simulink model "TSR_Scenario_002_cs"  (R2014b)
settings: Solver=ode5  SolverMode=SingleTasking  StartTime=0.0  StopTime=inf  FixedStep=1/100  RelTol=1e-3
PreLoadFcn:
  | mbxruntime.callbacks.PreLoadFcn(bdroot);
  | check_NUTS_defined;
  | 
  | assignin('base',['model_closed_' bdroot],false);
  | 
  | addpath('../includes_TSR/includes_TSR');
  | 
  | switch version('-release')
  | case {'2010a', '2010b', '2011a'}
  | addpath('../includes_TSR/ML2010b');
  | otherwise
  | addpath('../includes_TSR/ML2011b');
  | end
PostLoadFcn:
  | mbxruntime.callbacks.PostLoadFcn(bdroot);
InitFcn:
  | mbxruntime.callbacks.InitFcn(bdroot);;
  | 
  | addpath('..\includes_TSR');
StartFcn:
  | mbxruntime.callbacks.StartFcn(bdroot);
StopFcn:
  | mbxruntime.callbacks.StopFcn(bdroot);
model workspace: external: MAT-File .\TSR_Scenario_002_cs_hws.mat (data not in the file)
undefined symbols (not defined in the file or in its folder): InitImageOutputDir, mbxruntime, OrientationPitch, OrientationRoll, PositionX, PositionY, PositionZ, tabledata, warningInitialVelocity, x0
undefined symbols (not defined in the file): SteeringColumn, SteeringWheel, TSR_Scenario_002_cs_003e47b1b59594b6, TSR_Scenario_002_cs_023e87a31011dc74, TSR_Scenario_002_cs_048cb8409c90d9c6, TSR_Scenario_002_cs_106a0284aafa53e6, TSR_Scenario_002_cs_195b368d22a7f172, TSR_Scenario_002_cs_1e339fa5d680f213, TSR_Scenario_002_cs_26196a9fb104f950, TSR_Scenario_002_cs_261a709f6f453598, TSR_Scenario_002_cs_2ac3337370d0049d, TSR_Scenario_002_cs_2dc51e6a68b01b00, TSR_Scenario_002_cs_3460ff54d38ab2e2, TSR_Scenario_002_cs_42ea7d6e56bd6005, TSR_Scenario_002_cs_4dd419d6d2b56fc2, TSR_Scenario_002_cs_5316a21de09dff2f, TSR_Scenario_002_cs_538caacf3455966d, TSR_Scenario_002_cs_5b2cfdbcfc80811f, TSR_Scenario_002_cs_5ce0eafbb7a2dce7, TSR_Scenario_002_cs_62cdbf45c6f8824a, TSR_Scenario_002_cs_6bebc368eedff0bc, TSR_Scenario_002_cs_6d26481da4ed7e29, TSR_Scenario_002_cs_70c7e369ce6550e0, TSR_Scenario_002_cs_7a63051a1f311451, TSR_Scenario_002_cs_7d7dc8405f613c6d, TSR_Scenario_002_cs_7f65e296173485e8, TSR_Scenario_002_cs_87183cf6ff7bb4b6, TSR_Scenario_002_cs_8921b0da7ab80865, TSR_Scenario_002_cs_9495ce3a76763d1f, TSR_Scenario_002_cs_a679806a2fdc8099, TSR_Scenario_002_cs_Actros_1860_1_Path_pathUniqueID, TSR_Scenario_002_cs_Actros_2541_1_Path_pathUniqueID, TSR_Scenario_002_cs_Actros_2541_3_Path_pathUniqueID, TSR_Scenario_002_cs_Actros_2541_4_Path_pathUniqueID, TSR_Scenario_002_cs_adf24c93a9de8a4e, TSR_Scenario_002_cs_Audi_A8_1_Dynamics_Simple_initialPitch, TSR_Scenario_002_cs_Audi_A8_1_Dynamics_Simple_initialRoll, TSR_Scenario_002_cs_Audi_A8_1_Dynamics_Simple_initialX, TSR_Scenario_002_cs_Audi_A8_1_Dynamics_Simple_initialY, TSR_Scenario_002_cs_Audi_A8_1_Dynamics_Simple_initialYaw, TSR_Scenario_002_cs_Audi_A8_1_Dynamics_Simple_initialZ, TSR_Scenario_002_cs_b136c6ccb55f77db, TSR_Scenario_002_cs_ba4f809714c282b7, TSR_Scenario_002_cs_BMW_X5_1_Path_pathUniqueID, TSR_Scenario_002_cs_BMW_X5_1_SpeedProfile_speedProfileUniqueID, TSR_Scenario_002_cs_BMW_X5_2_Path_pathUniqueID, TSR_Scenario_002_cs_BMW_X5_2_SpeedProfile_speedProfileUniqueID, TSR_Scenario_002_cs_Citroen_C3_1_Path_pathUniqueID, TSR_Scenario_002_cs_Citroen_C3_2_Path_pathUniqueID, TSR_Scenario_002_cs_d8f275339b7082cf, TSR_Scenario_002_cs_Daf_95_1_Path_pathUniqueID, TSR_Scenario_002_cs_Daf_95_1_SpeedProfile_speedProfileUniqueID, TSR_Scenario_002_cs_dc019741510ce2f2, TSR_Scenario_002_cs_fdbc8aabe460b27c, TSR_Scenario_002_cs_Fiat_Bravo_1_Path_pathUniqueID, TSR_Scenario_002_cs_Ford_Fiesta_1_Path_pathUniqueID, TSR_Scenario_002_cs_Honda_Pan_European_1_Path_pathUniqueID, TSR_Scenario_002_cs_Mazda_RX8_1_Path_pathUniqueID, TSR_Scenario_002_cs_Nissan_Cabstar_1_Path_pathUniqueID, TSR_Scenario_002_cs_Nissan_Cabstar_2_Path_pathUniqueID ... (+9)
libraries: simulink_extras x82, simulink x23, PreScanSimulinkLibrary x11
(part 10 of 39)

== system TSR_Scenario_002_cs/HighwayOverhang_11 ==
  note: Resources
      |
      | 1: InformationSign\MatrixSign_GreenArrow.png: MatrixSign GreenArrow
      | 2: InformationSign\Empty.jpeg: Empty
      | 3: InformationSign\SEARCH_Logo.png: SEARCH Logo
      | 4: InformationSign\z274-50_black_full.png: z274-50 black full
      | 5: InformationSign\z274-51_black_full.png: z274-51 black full
      | 6: InformationSign\z274-52_black_full.png: z274-52 black full
      | 7: InformationSign\z274-53_black_full.png: z274-53 black full
      | 8: InformationSign\z274-54_black_full.png: z274-54 black full
      | 9: InformationSign\z274-55_black_full.png: z274-55 black full
      | 10: InformationSign\z274-56_black_full.png: z274-56 black full
      | 11: InformationSign\z274-57_black_full.png: z274-57 black full
      | 12: InformationSign\z274-58_black_full.png: z274-58 black full
      | 13: InformationSign\z274-59_black_full.png: z274-59 black full
      | 14: InformationSign\z274-60_black_full.png: z274-60 black full
      | 15: InformationSign\z274-61_black_full.png: z274-61 black full
      | 16: InformationSign\z274-62_black_full.png: z274-62 black full
      | 17: InformationSign\z274-63_black_full.png: z274-63 black full
  Ground_{1..4} (4 alike) : Ground
  VISUMatrixSignLights_Mux : Subsystem  Tag=mux/VisuMatrixSignLights  mask(PreScan User Interface: VisuMatrixSignLights){}
      mask help:
      | The VisuMatrixSignLights block provides a way to switch the lights on the matrix sign board on or off
      |
      | For more information, please click Help.
      mask Help: eval('openHelp(732)')
  VISUMatrixSign_Mux : Subsystem  Tag=mux/MatrixSign_v2  mask(PreScan User Interface: VisuMatrixSign){}
      mask help:
      | The VisuMatrixSign block provides a way to adapt the texture of the plates connected to an overhang, based on Resource IDs of the texture files.
      |
      | For more information, please click Help.
      settings: DeleteFcn=PreScanBlockDeleteFcn;
      mask Help: eval('openHelp(733)')
  VISUMatrixSign_HighwayOverhang_11 : Outport  Tag=outport/VisuMatrixSign  SampleTime=1/100
  VISUMatrixSignLights_HighwayOverhang_11 : Outport  Tag=outport/VisuMatrixSignLights  Port=2  SampleTime=1/100
  wires:
  VISUMatrixSign_Mux/1(MatrixSigns) -> VISUMatrixSign_HighwayOverhang_11/1
  VISUMatrixSignLights_Mux/1(VISUMatrixSignLights_HighwayOverhang_11) -> VISUMatrixSignLights_HighwayOverhang_11/1
  Ground_1/1 -> VISUMatrixSignLights_Mux/1(MatrixSign_10)
  Ground_2/1 -> VISUMatrixSignLights_Mux/2(MatrixSign_49)
  Ground_3/1 -> VISUMatrixSign_Mux/1(MatrixSign_10)
  Ground_4/1 -> VISUMatrixSign_Mux/2(MatrixSign_49)

== system TSR_Scenario_002_cs/HighwayOverhang_12 ==
  note: Resources
      |
      | 1: InformationSign\MatrixSign_GreenArrow.png: MatrixSign GreenArrow
      | 2: InformationSign\Empty.jpeg: Empty
      | 3: InformationSign\SEARCH_Logo.png: SEARCH Logo
      | 4: InformationSign\z274-50_black_full.png: z274-50 black full
      | 5: InformationSign\z274-51_black_full.png: z274-51 black full
      | 6: InformationSign\z274-52_black_full.png: z274-52 black full
      | 7: InformationSign\z274-53_black_full.png: z274-53 black full
      | 8: InformationSign\z274-54_black_full.png: z274-54 black full
      | 9: InformationSign\z274-55_black_full.png: z274-55 black full
      | 10: InformationSign\z274-56_black_full.png: z274-56 black full
      | 11: InformationSign\z274-57_black_full.png: z274-57 black full
      | 12: InformationSign\z274-58_black_full.png: z274-58 black full
      | 13: InformationSign\z274-59_black_full.png: z274-59 black full
      | 14: InformationSign\z274-60_black_full.png: z274-60 black full
      | 15: InformationSign\z274-61_black_full.png: z274-61 black full
      | 16: InformationSign\z274-62_black_full.png: z274-62 black full
      | 17: InformationSign\z274-63_black_full.png: z274-63 black full
  Ground_{1..4} (4 alike) : Ground
  VISUMatrixSignLights_Mux : Subsystem  Tag=mux/VisuMatrixSignLights  mask(PreScan User Interface: VisuMatrixSignLights){}
      mask help:
      | The VisuMatrixSignLights block provides a way to switch the lights on the matrix sign board on or off
      |
      | For more information, please click Help.
      mask Help: eval('openHelp(732)')
  VISUMatrixSign_Mux : Subsystem  Tag=mux/MatrixSign_v2  mask(PreScan User Interface: VisuMatrixSign){}
      mask help:
      | The VisuMatrixSign block provides a way to adapt the texture of the plates connected to an overhang, based on Resource IDs of the texture files.
      |
      | For more information, please click Help.
      settings: DeleteFcn=PreScanBlockDeleteFcn;
      mask Help: eval('openHelp(733)')
  VISUMatrixSign_HighwayOverhang_12 : Outport  Tag=outport/VisuMatrixSign  SampleTime=1/100
  VISUMatrixSignLights_HighwayOverhang_12 : Outport  Tag=outport/VisuMatrixSignLights  Port=2  SampleTime=1/100
  wires:
  VISUMatrixSign_Mux/1(MatrixSigns) -> VISUMatrixSign_HighwayOverhang_12/1
  VISUMatrixSignLights_Mux/1(VISUMatrixSignLights_HighwayOverhang_12) -> VISUMatrixSignLights_HighwayOverhang_12/1
  Ground_1/1 -> VISUMatrixSignLights_Mux/1(MatrixSign_21)
  Ground_2/1 -> VISUMatrixSignLights_Mux/2(MatrixSign_22)
  Ground_3/1 -> VISUMatrixSign_Mux/1(MatrixSign_21)
  Ground_4/1 -> VISUMatrixSign_Mux/2(MatrixSign_22)

== system TSR_Scenario_002_cs/HighwayOverhang_13 ==
  note: Resources
      |
      | 1: InformationSign\MatrixSign_GreenArrow.png: MatrixSign GreenArrow
      | 2: InformationSign\Empty.jpeg: Empty
      | 3: InformationSign\SEARCH_Logo.png: SEARCH Logo
      | 4: InformationSign\z274-50_black_full.png: z274-50 black full
      | 5: InformationSign\z274-51_black_full.png: z274-51 black full
      | 6: InformationSign\z274-52_black_full.png: z274-52 black full
      | 7: InformationSign\z274-53_black_full.png: z274-53 black full
      | 8: InformationSign\z274-54_black_full.png: z274-54 black full
      | 9: InformationSign\z274-55_black_full.png: z274-55 black full
      | 10: InformationSign\z274-56_black_full.png: z274-56 black full
      | 11: InformationSign\z274-57_black_full.png: z274-57 black full
      | 12: InformationSign\z274-58_black_full.png: z274-58 black full
      | 13: InformationSign\z274-59_black_full.png: z274-59 black full
      | 14: InformationSign\z274-60_black_full.png: z274-60 black full
      | 15: InformationSign\z274-61_black_full.png: z274-61 black full
      | 16: InformationSign\z274-62_black_full.png: z274-62 black full
      | 17: InformationSign\z274-63_black_full.png: z274-63 black full
  Ground_{1..4} (4 alike) : Ground
  VISUMatrixSignLights_Mux : Subsystem  Tag=mux/VisuMatrixSignLights  mask(PreScan User Interface: VisuMatrixSignLights){}
      mask help:
      | The VisuMatrixSignLights block provides a way to switch the lights on the matrix sign board on or off
      |
      | For more information, please click Help.
      mask Help: eval('openHelp(732)')
  VISUMatrixSign_Mux : Subsystem  Tag=mux/MatrixSign_v2  mask(PreScan User Interface: VisuMatrixSign){}
      mask help:
      | The VisuMatrixSign block provides a way to adapt the texture of the plates connected to an overhang, based on Resource IDs of the texture files.
      |
      | For more information, please click Help.
      settings: DeleteFcn=PreScanBlockDeleteFcn;
      mask Help: eval('openHelp(733)')
  VISUMatrixSign_HighwayOverhang_13 : Outport  Tag=outport/VisuMatrixSign  SampleTime=1/100
  VISUMatrixSignLights_HighwayOverhang_13 : Outport  Tag=outport/VisuMatrixSignLights  Port=2  SampleTime=1/100
  wires:
  VISUMatrixSign_Mux/1(MatrixSigns) -> VISUMatrixSign_HighwayOverhang_13/1
  VISUMatrixSignLights_Mux/1(VISUMatrixSignLights_HighwayOverhang_13) -> VISUMatrixSignLights_HighwayOverhang_13/1
  Ground_1/1 -> VISUMatrixSignLights_Mux/1(MatrixSign_3)
  Ground_2/1 -> VISUMatrixSignLights_Mux/2(MatrixSign_44)
  Ground_3/1 -> VISUMatrixSign_Mux/1(MatrixSign_3)
  Ground_4/1 -> VISUMatrixSign_Mux/2(MatrixSign_44)

== system TSR_Scenario_002_cs/HighwayOverhang_14 ==
  note: Resources
      |
      | 1: InformationSign\MatrixSign_GreenArrow.png: MatrixSign GreenArrow
      | 2: InformationSign\Empty.jpeg: Empty
      | 3: InformationSign\SEARCH_Logo.png: SEARCH Logo
      | 4: InformationSign\z274-50_black_full.png: z274-50 black full
      | 5: InformationSign\z274-51_black_full.png: z274-51 black full
      | 6: InformationSign\z274-52_black_full.png: z274-52 black full
      | 7: InformationSign\z274-53_black_full.png: z274-53 black full
      | 8: InformationSign\z274-54_black_full.png: z274-54 black full
      | 9: InformationSign\z274-55_black_full.png: z274-55 black full
      | 10: InformationSign\z274-56_black_full.png: z274-56 black full
      | 11: InformationSign\z274-57_black_full.png: z274-57 black full
      | 12: InformationSign\z274-58_black_full.png: z274-58 black full
      | 13: InformationSign\z274-59_black_full.png: z274-59 black full
      | 14: InformationSign\z274-60_black_full.png: z274-60 black full
      | 15: InformationSign\z274-61_black_full.png: z274-61 black full
      | 16: InformationSign\z274-62_black_full.png: z274-62 black full
      | 17: InformationSign\z274-63_black_full.png: z274-63 black full
  Ground_{1..4} (4 alike) : Ground
  VISUMatrixSignLights_Mux : Subsystem  Tag=mux/VisuMatrixSignLights  mask(PreScan User Interface: VisuMatrixSignLights){}
      mask help:
      | The VisuMatrixSignLights block provides a way to switch the lights on the matrix sign board on or off
      |
      | For more information, please click Help.
      mask Help: eval('openHelp(732)')
  VISUMatrixSign_Mux : Subsystem  Tag=mux/MatrixSign_v2  mask(PreScan User Interface: VisuMatrixSign){}
      mask help:
      | The VisuMatrixSign block provides a way to adapt the texture of the plates connected to an overhang, based on Resource IDs of the texture files.
      |
      | For more information, please click Help.
      settings: DeleteFcn=PreScanBlockDeleteFcn;
      mask Help: eval('openHelp(733)')
  VISUMatrixSign_HighwayOverhang_14 : Outport  Tag=outport/VisuMatrixSign  SampleTime=1/100
  VISUMatrixSignLights_HighwayOverhang_14 : Outport  Tag=outport/VisuMatrixSignLights  Port=2  SampleTime=1/100
  wires:
  VISUMatrixSign_Mux/1(MatrixSigns) -> VISUMatrixSign_HighwayOverhang_14/1
  VISUMatrixSignLights_Mux/1(VISUMatrixSignLights_HighwayOverhang_14) -> VISUMatrixSignLights_HighwayOverhang_14/1
  Ground_1/1 -> VISUMatrixSignLights_Mux/1(MatrixSign_27)
  Ground_2/1 -> VISUMatrixSignLights_Mux/2(MatrixSign_28)
  Ground_3/1 -> VISUMatrixSign_Mux/1(MatrixSign_27)
  Ground_4/1 -> VISUMatrixSign_Mux/2(MatrixSign_28)

== system TSR_Scenario_002_cs/HighwayOverhang_15 ==
  note: Resources
      |
      | 1: InformationSign\MatrixSign_GreenArrow.png: MatrixSign GreenArrow
      | 2: InformationSign\Empty.jpeg: Empty
      | 3: InformationSign\SEARCH_Logo.png: SEARCH Logo
      | 4: InformationSign\z274-50_black_full.png: z274-50 black full
      | 5: InformationSign\z274-51_black_full.png: z274-51 black full
      | 6: InformationSign\z274-52_black_full.png: z274-52 black full
      | 7: InformationSign\z274-53_black_full.png: z274-53 black full
      | 8: InformationSign\z274-54_black_full.png: z274-54 black full
      | 9: InformationSign\z274-55_black_full.png: z274-55 black full
      | 10: InformationSign\z274-56_black_full.png: z274-56 black full
      | 11: InformationSign\z274-57_black_full.png: z274-57 black full
      | 12: InformationSign\z274-58_black_full.png: z274-58 black full
      | 13: InformationSign\z274-59_black_full.png: z274-59 black full
      | 14: InformationSign\z274-60_black_full.png: z274-60 black full
      | 15: InformationSign\z274-61_black_full.png: z274-61 black full
      | 16: InformationSign\z274-62_black_full.png: z274-62 black full
      | 17: InformationSign\z274-63_black_full.png: z274-63 black full
  Ground_{1..4} (4 alike) : Ground
  VISUMatrixSignLights_Mux : Subsystem  Tag=mux/VisuMatrixSignLights  mask(PreScan User Interface: VisuMatrixSignLights){}
      mask help:
      | The VisuMatrixSignLights block provides a way to switch the lights on the matrix sign board on or off
      |
      | For more information, please click Help.
      mask Help: eval('openHelp(732)')
  VISUMatrixSign_Mux : Subsystem  Tag=mux/MatrixSign_v2  mask(PreScan User Interface: VisuMatrixSign){}
      mask help:
      | The VisuMatrixSign block provides a way to adapt the texture of the plates connected to an overhang, based on Resource IDs of the texture files.
      |
      | For more information, please click Help.
      settings: DeleteFcn=PreScanBlockDeleteFcn;
      mask Help: eval('openHelp(733)')
  VISUMatrixSign_HighwayOverhang_15 : Outport  Tag=outport/VisuMatrixSign  SampleTime=1/100
  VISUMatrixSignLights_HighwayOverhang_15 : Outport  Tag=outport/VisuMatrixSignLights  Port=2  SampleTime=1/100
  wires:
  VISUMatrixSign_Mux/1(MatrixSigns) -> VISUMatrixSign_HighwayOverhang_15/1
  VISUMatrixSignLights_Mux/1(VISUMatrixSignLights_HighwayOverhang_15) -> VISUMatrixSignLights_HighwayOverhang_15/1
  Ground_1/1 -> VISUMatrixSignLights_Mux/1(MatrixSign_46)
  Ground_2/1 -> VISUMatrixSignLights_Mux/2(MatrixSign_5)
  Ground_3/1 -> VISUMatrixSign_Mux/1(MatrixSign_5)
  Ground_4/1 -> VISUMatrixSign_Mux/2(MatrixSign_46)

== system TSR_Scenario_002_cs/HighwayOverhang_16 ==
  note: Resources
      |
      | 1: InformationSign\MatrixSign_GreenArrow.png: MatrixSign GreenArrow
      | 2: InformationSign\Empty.jpeg: Empty
      | 3: InformationSign\SEARCH_Logo.png: SEARCH Logo
      | 4: InformationSign\z274-50_black_full.png: z274-50 black full
      | 5: InformationSign\z274-51_black_full.png: z274-51 black full
      | 6: InformationSign\z274-52_black_full.png: z274-52 black full
      | 7: InformationSign\z274-53_black_full.png: z274-53 black full
      | 8: InformationSign\z274-54_black_full.png: z274-54 black full
      | 9: InformationSign\z274-55_black_full.png: z274-55 black full
      | 10: InformationSign\z274-56_black_full.png: z274-56 black full
      | 11: InformationSign\z274-57_black_full.png: z274-57 black full
      | 12: InformationSign\z274-58_black_full.png: z274-58 black full
      | 13: InformationSign\z274-59_black_full.png: z274-59 black full
      | 14: InformationSign\z274-60_black_full.png: z274-60 black full
      | 15: InformationSign\z274-61_black_full.png: z274-61 black full
      | 16: InformationSign\z274-62_black_full.png: z274-62 black full
      | 17: InformationSign\z274-63_black_full.png: z274-63 black full
  Ground_{1..4} (4 alike) : Ground
  VISUMatrixSignLights_Mux : Subsystem  Tag=mux/VisuMatrixSignLights  mask(PreScan User Interface: VisuMatrixSignLights){}
      mask help:
      | The VisuMatrixSignLights block provides a way to switch the lights on the matrix sign board on or off
      |
      | For more information, please click Help.
      mask Help: eval('openHelp(732)')
  VISUMatrixSign_Mux : Subsystem  Tag=mux/MatrixSign_v2  mask(PreScan User Interface: VisuMatrixSign){}
      mask help:
      | The VisuMatrixSign block provides a way to adapt the texture of the plates connected to an overhang, based on Resource IDs of the texture files.
      |
      | For more information, please click Help.
      settings: DeleteFcn=PreScanBlockDeleteFcn;
      mask Help: eval('openHelp(733)')
  VISUMatrixSign_HighwayOverhang_16 : Outport  Tag=outport/VisuMatrixSign  SampleTime=1/100
  VISUMatrixSignLights_HighwayOverhang_16 : Outport  Tag=outport/VisuMatrixSignLights  Port=2  SampleTime=1/100
  wires:
  VISUMatrixSign_Mux/1(MatrixSigns) -> VISUMatrixSign_HighwayOverhang_16/1
  VISUMatrixSignLights_Mux/1(VISUMatrixSignLights_HighwayOverhang_16) -> VISUMatrixSignLights_HighwayOverhang_16/1
  Ground_1/1 -> VISUMatrixSignLights_Mux/1(MatrixSign_29)
  Ground_2/1 -> VISUMatrixSignLights_Mux/2(MatrixSign_30)
  Ground_3/1 -> VISUMatrixSign_Mux/1(MatrixSign_29)
  Ground_4/1 -> VISUMatrixSign_Mux/2(MatrixSign_30)

== system TSR_Scenario_002_cs/HighwayOverhang_17 ==
  note: Resources
      |
      | 1: InformationSign\MatrixSign_GreenArrow.png: MatrixSign GreenArrow
      | 2: InformationSign\Empty.jpeg: Empty
      | 3: InformationSign\SEARCH_Logo.png: SEARCH Logo
      | 4: InformationSign\z274-50_black_full.png: z274-50 black full
      | 5: InformationSign\z274-51_black_full.png: z274-51 black full
      | 6: InformationSign\z274-52_black_full.png: z274-52 black full
      | 7: InformationSign\z274-53_black_full.png: z274-53 black full
      | 8: InformationSign\z274-54_black_full.png: z274-54 black full
      | 9: InformationSign\z274-55_black_full.png: z274-55 black full
      | 10: InformationSign\z274-56_black_full.png: z274-56 black full
      | 11: InformationSign\z274-57_black_full.png: z274-57 black full
      | 12: InformationSign\z274-58_black_full.png: z274-58 black full
      | 13: InformationSign\z274-59_black_full.png: z274-59 black full
      | 14: InformationSign\z274-60_black_full.png: z274-60 black full
      | 15: InformationSign\z274-61_black_full.png: z274-61 black full
      | 16: InformationSign\z274-62_black_full.png: z274-62 black full
      | 17: InformationSign\z274-63_black_full.png: z274-63 black full
  Ground_{1..4} (4 alike) : Ground
  VISUMatrixSignLights_Mux : Subsystem  Tag=mux/VisuMatrixSignLights  mask(PreScan User Interface: VisuMatrixSignLights){}
      mask help:
      | The VisuMatrixSignLights block provides a way to switch the lights on the matrix sign board on or off
      |
      | For more information, please click Help.
      mask Help: eval('openHelp(732)')
  VISUMatrixSign_Mux : Subsystem  Tag=mux/MatrixSign_v2  mask(PreScan User Interface: VisuMatrixSign){}
      mask help:
      | The VisuMatrixSign block provides a way to adapt the texture of the plates connected to an overhang, based on Resource IDs of the texture files.
      |
      | For more information, please click Help.
      settings: DeleteFcn=PreScanBlockDeleteFcn;
      mask Help: eval('openHelp(733)')
  VISUMatrixSign_HighwayOverhang_17 : Outport  Tag=outport/VisuMatrixSign  SampleTime=1/100
  VISUMatrixSignLights_HighwayOverhang_17 : Outport  Tag=outport/VisuMatrixSignLights  Port=2  SampleTime=1/100
  wires:
  VISUMatrixSign_Mux/1(MatrixSigns) -> VISUMatrixSign_HighwayOverhang_17/1
  VISUMatrixSignLights_Mux/1(VISUMatrixSignLights_HighwayOverhang_17) -> VISUMatrixSignLights_HighwayOverhang_17/1
  Ground_1/1 -> VISUMatrixSignLights_Mux/1(MatrixSign_51)
  Ground_2/1 -> VISUMatrixSignLights_Mux/2(MatrixSign_7)
  Ground_3/1 -> VISUMatrixSign_Mux/1(MatrixSign_7)
  Ground_4/1 -> VISUMatrixSign_Mux/2(MatrixSign_51)

== system TSR_Scenario_002_cs/HighwayOverhang_18 ==
  note: Resources
      |
      | 1: InformationSign\MatrixSign_GreenArrow.png: MatrixSign GreenArrow
      | 2: InformationSign\Empty.jpeg: Empty
      | 3: InformationSign\SEARCH_Logo.png: SEARCH Logo
      | 4: InformationSign\z274-50_black_full.png: z274-50 black full
      | 5: InformationSign\z274-51_black_full.png: z274-51 black full
      | 6: InformationSign\z274-52_black_full.png: z274-52 black full
      | 7: InformationSign\z274-53_black_full.png: z274-53 black full
      | 8: InformationSign\z274-54_black_full.png: z274-54 black full
      | 9: InformationSign\z274-55_black_full.png: z274-55 black full
      | 10: InformationSign\z274-56_black_full.png: z274-56 black full
      | 11: InformationSign\z274-57_black_full.png: z274-57 black full
      | 12: InformationSign\z274-58_black_full.png: z274-58 black full
      | 13: InformationSign\z274-59_black_full.png: z274-59 black full
      | 14: InformationSign\z274-60_black_full.png: z274-60 black full
      | 15: InformationSign\z274-61_black_full.png: z274-61 black full
      | 16: InformationSign\z274-62_black_full.png: z274-62 black full
      | 17: InformationSign\z274-63_black_full.png: z274-63 black full
  Ground_{1..4} (4 alike) : Ground
  VISUMatrixSignLights_Mux : Subsystem  Tag=mux/VisuMatrixSignLights  mask(PreScan User Interface: VisuMatrixSignLights){}
      mask help:
      | The VisuMatrixSignLights block provides a way to switch the lights on the matrix sign board on or off
      |
      | For more information, please click Help.
      mask Help: eval('openHelp(732)')
  VISUMatrixSign_Mux : Subsystem  Tag=mux/MatrixSign_v2  mask(PreScan User Interface: VisuMatrixSign){}
      mask help:
      | The VisuMatrixSign block provides a way to adapt the texture of the plates connected to an overhang, based on Resource IDs of the texture files.
      |
      | For more information, please click Help.
      settings: DeleteFcn=PreScanBlockDeleteFcn;
      mask Help: eval('openHelp(733)')
  VISUMatrixSign_HighwayOverhang_18 : Outport  Tag=outport/VisuMatrixSign  SampleTime=1/100
  VISUMatrixSignLights_HighwayOverhang_18 : Outport  Tag=outport/VisuMatrixSignLights  Port=2  SampleTime=1/100
  wires:
  VISUMatrixSign_Mux/1(MatrixSigns) -> VISUMatrixSign_HighwayOverhang_18/1
  VISUMatrixSignLights_Mux/1(VISUMatrixSignLights_HighwayOverhang_18) -> VISUMatrixSignLights_HighwayOverhang_18/1
  Ground_1/1 -> VISUMatrixSignLights_Mux/1(MatrixSign_31)
  Ground_2/1 -> VISUMatrixSignLights_Mux/2(MatrixSign_32)
  Ground_3/1 -> VISUMatrixSign_Mux/1(MatrixSign_31)
  Ground_4/1 -> VISUMatrixSign_Mux/2(MatrixSign_32)

== system TSR_Scenario_002_cs/HighwayOverhang_19 ==
  note: Resources
      |
      | 1: InformationSign\MatrixSign_GreenArrow.png: MatrixSign GreenArrow
      | 2: InformationSign\Empty.jpeg: Empty
      | 3: InformationSign\SEARCH_Logo.png: SEARCH Logo
      | 4: InformationSign\z274-50_black_full.png: z274-50 black full
      | 5: InformationSign\z274-51_black_full.png: z274-51 black full
      | 6: InformationSign\z274-52_black_full.png: z274-52 black full
      | 7: InformationSign\z274-53_black_full.png: z274-53 black full
      | 8: InformationSign\z274-54_black_full.png: z274-54 black full
      | 9: InformationSign\z274-55_black_full.png: z274-55 black full
      | 10: InformationSign\z274-56_black_full.png: z274-56 black full
      | 11: InformationSign\z274-57_black_full.png: z274-57 black full
      | 12: InformationSign\z274-58_black_full.png: z274-58 black full
      | 13: InformationSign\z274-59_black_full.png: z274-59 black full
      | 14: InformationSign\z274-60_black_full.png: z274-60 black full
      | 15: InformationSign\z274-61_black_full.png: z274-61 black full
      | 16: InformationSign\z274-62_black_full.png: z274-62 black full
      | 17: InformationSign\z274-63_black_full.png: z274-63 black full
  Ground_{1..4} (4 alike) : Ground
  VISUMatrixSignLights_Mux : Subsystem  Tag=mux/VisuMatrixSignLights  mask(PreScan User Interface: VisuMatrixSignLights){}
      mask help:
      | The VisuMatrixSignLights block provides a way to switch the lights on the matrix sign board on or off
      |
      | For more information, please click Help.
      mask Help: eval('openHelp(732)')
  VISUMatrixSign_Mux : Subsystem  Tag=mux/MatrixSign_v2  mask(PreScan User Interface: VisuMatrixSign){}
      mask help:
      | The VisuMatrixSign block provides a way to adapt the texture of the plates connected to an overhang, based on Resource IDs of the texture files.
      |
      | For more information, please click Help.
      settings: DeleteFcn=PreScanBlockDeleteFcn;
      mask Help: eval('openHelp(733)')
  VISUMatrixSign_HighwayOverhang_19 : Outport  Tag=outport/VisuMatrixSign  SampleTime=1/100
  VISUMatrixSignLights_HighwayOverhang_19 : Outport  Tag=outport/VisuMatrixSignLights  Port=2  SampleTime=1/100
  wires:
  VISUMatrixSign_Mux/1(MatrixSigns) -> VISUMatrixSign_HighwayOverhang_19/1
  VISUMatrixSignLights_Mux/1(VISUMatrixSignLights_HighwayOverhang_19) -> VISUMatrixSignLights_HighwayOverhang_19/1
  Ground_1/1 -> VISUMatrixSignLights_Mux/1(MatrixSign_52)
  Ground_2/1 -> VISUMatrixSignLights_Mux/2(MatrixSign_9)
  Ground_3/1 -> VISUMatrixSign_Mux/1(MatrixSign_9)
  Ground_4/1 -> VISUMatrixSign_Mux/2(MatrixSign_52)

== system TSR_Scenario_002_cs/HighwayOverhang_2 ==
  note: Resources
      |
      | 1: InformationSign\MatrixSign_GreenArrow.png: MatrixSign GreenArrow
      | 2: InformationSign\Empty.jpeg: Empty
      | 3: InformationSign\SEARCH_Logo.png: SEARCH Logo
      | 4: InformationSign\z274-50_black_full.png: z274-50 black full
      | 5: InformationSign\z274-51_black_full.png: z274-51 black full
      | 6: InformationSign\z274-52_black_full.png: z274-52 black full
      | 7: InformationSign\z274-53_black_full.png: z274-53 black full
      | 8: InformationSign\z274-54_black_full.png: z274-54 black full
      | 9: InformationSign\z274-55_black_full.png: z274-55 black full
      | 10: InformationSign\z274-56_black_full.png: z274-56 black full
      | 11: InformationSign\z274-57_black_full.png: z274-57 black full
      | 12: InformationSign\z274-58_black_full.png: z274-58 black full
      | 13: InformationSign\z274-59_black_full.png: z274-59 black full
      | 14: InformationSign\z274-60_black_full.png: z274-60 black full
      | 15: InformationSign\z274-61_black_full.png: z274-61 black full
      | 16: InformationSign\z274-62_black_full.png: z274-62 black full
      | 17: InformationSign\z274-63_black_full.png: z274-63 black full
  Ground_{1..4} (4 alike) : Ground
  VISUMatrixSignLights_Mux : Subsystem  Tag=mux/VisuMatrixSignLights  mask(PreScan User Interface: VisuMatrixSignLights){}
      mask help:
      | The VisuMatrixSignLights block provides a way to switch the lights on the matrix sign board on or off
      |
      | For more information, please click Help.
      mask Help: eval('openHelp(732)')
  VISUMatrixSign_Mux : Subsystem  Tag=mux/MatrixSign_v2  mask(PreScan User Interface: VisuMatrixSign){}
      mask help:
      | The VisuMatrixSign block provides a way to adapt the texture of the plates connected to an overhang, based on Resource IDs of the texture files.
      |
      | For more information, please click Help.
      settings: DeleteFcn=PreScanBlockDeleteFcn;
      mask Help: eval('openHelp(733)')
  VISUMatrixSign_HighwayOverhang_2 : Outport  Tag=outport/VisuMatrixSign  SampleTime=1/100
  VISUMatrixSignLights_HighwayOverhang_2 : Outport  Tag=outport/VisuMatrixSignLights  Port=2  SampleTime=1/100
  wires:
  VISUMatrixSign_Mux/1(MatrixSigns) -> VISUMatrixSign_HighwayOverhang_2/1
  VISUMatrixSignLights_Mux/1(VISUMatrixSignLights_HighwayOverhang_2) -> VISUMatrixSignLights_HighwayOverhang_2/1
  Ground_1/1 -> VISUMatrixSignLights_Mux/1(MatrixSign_14)
  Ground_2/1 -> VISUMatrixSignLights_Mux/2(MatrixSign_2)
  Ground_3/1 -> VISUMatrixSign_Mux/1(MatrixSign_14)
  Ground_4/1 -> VISUMatrixSign_Mux/2(MatrixSign_2)

== system TSR_Scenario_002_cs/HighwayOverhang_20 ==
  note: Resources
      |
      | 1: InformationSign\MatrixSign_GreenArrow.png: MatrixSign GreenArrow
      | 2: InformationSign\Empty.jpeg: Empty
      | 3: InformationSign\SEARCH_Logo.png: SEARCH Logo
      | 4: InformationSign\z274-50_black_full.png: z274-50 black full
      | 5: InformationSign\z274-51_black_full.png: z274-51 black full
      | 6: InformationSign\z274-52_black_full.png: z274-52 black full
      | 7: InformationSign\z274-53_black_full.png: z274-53 black full
      | 8: InformationSign\z274-54_black_full.png: z274-54 black full
      | 9: InformationSign\z274-55_black_full.png: z274-55 black full
      | 10: InformationSign\z274-56_black_full.png: z274-56 black full
      | 11: InformationSign\z274-57_black_full.png: z274-57 black full
      | 12: InformationSign\z274-58_black_full.png: z274-58 black full
      | 13: InformationSign\z274-59_black_full.png: z274-59 black full
      | 14: InformationSign\z274-60_black_full.png: z274-60 black full
      | 15: InformationSign\z274-61_black_full.png: z274-61 black full
      | 16: InformationSign\z274-62_black_full.png: z274-62 black full
      | 17: InformationSign\z274-63_black_full.png: z274-63 black full
  Ground_{1..4} (4 alike) : Ground
  VISUMatrixSignLights_Mux : Subsystem  Tag=mux/VisuMatrixSignLights  mask(PreScan User Interface: VisuMatrixSignLights){}
      mask help:
      | The VisuMatrixSignLights block provides a way to switch the lights on the matrix sign board on or off
      |
      | For more information, please click Help.
      mask Help: eval('openHelp(732)')
  VISUMatrixSign_Mux : Subsystem  Tag=mux/MatrixSign_v2  mask(PreScan User Interface: VisuMatrixSign){}
      mask help:
      | The VisuMatrixSign block provides a way to adapt the texture of the plates connected to an overhang, based on Resource IDs of the texture files.
      |
      | For more information, please click Help.
      settings: DeleteFcn=PreScanBlockDeleteFcn;
      mask Help: eval('openHelp(733)')
  VISUMatrixSign_HighwayOverhang_20 : Outport  Tag=outport/VisuMatrixSign  SampleTime=1/100
  VISUMatrixSignLights_HighwayOverhang_20 : Outport  Tag=outport/VisuMatrixSignLights  Port=2  SampleTime=1/100
  wires:
  VISUMatrixSign_Mux/1(MatrixSigns) -> VISUMatrixSign_HighwayOverhang_20/1
  VISUMatrixSignLights_Mux/1(VISUMatrixSignLights_HighwayOverhang_20) -> VISUMatrixSignLights_HighwayOverhang_20/1
  Ground_1/1 -> VISUMatrixSignLights_Mux/1(MatrixSign_33)
  Ground_2/1 -> VISUMatrixSignLights_Mux/2(MatrixSign_34)
  Ground_3/1 -> VISUMatrixSign_Mux/1(MatrixSign_33)
  Ground_4/1 -> VISUMatrixSign_Mux/2(MatrixSign_34)

== system TSR_Scenario_002_cs/HighwayOverhang_21 ==
  note: Resources
      |
      | 1: InformationSign\MatrixSign_GreenArrow.png: MatrixSign GreenArrow
      | 2: InformationSign\Empty.jpeg: Empty
      | 3: InformationSign\SEARCH_Logo.png: SEARCH Logo
      | 4: InformationSign\z274-50_black_full.png: z274-50 black full
      | 5: InformationSign\z274-51_black_full.png: z274-51 black full
      | 6: InformationSign\z274-52_black_full.png: z274-52 black full
      | 7: InformationSign\z274-53_black_full.png: z274-53 black full
      | 8: InformationSign\z274-54_black_full.png: z274-54 black full
      | 9: InformationSign\z274-55_black_full.png: z274-55 black full
      | 10: InformationSign\z274-56_black_full.png: z274-56 black full
      | 11: InformationSign\z274-57_black_full.png: z274-57 black full
      | 12: InformationSign\z274-58_black_full.png: z274-58 black full
      | 13: InformationSign\z274-59_black_full.png: z274-59 black full
      | 14: InformationSign\z274-60_black_full.png: z274-60 black full
      | 15: InformationSign\z274-61_black_full.png: z274-61 black full
      | 16: InformationSign\z274-62_black_full.png: z274-62 black full
      | 17: InformationSign\z274-63_black_full.png: z274-63 black full
  Ground_{1..4} (4 alike) : Ground
  VISUMatrixSignLights_Mux : Subsystem  Tag=mux/VisuMatrixSignLights  mask(PreScan User Interface: VisuMatrixSignLights){}
      mask help:
      | The VisuMatrixSignLights block provides a way to switch the lights on the matrix sign board on or off
      |
      | For more information, please click Help.
      mask Help: eval('openHelp(732)')
  VISUMatrixSign_Mux : Subsystem  Tag=mux/MatrixSign_v2  mask(PreScan User Interface: VisuMatrixSign){}
      mask help:
      | The VisuMatrixSign block provides a way to adapt the texture of the plates connected to an overhang, based on Resource IDs of the texture files.
      |
      | For more information, please click Help.
      settings: DeleteFcn=PreScanBlockDeleteFcn;
      mask Help: eval('openHelp(733)')
  VISUMatrixSign_HighwayOverhang_21 : Outport  Tag=outport/VisuMatrixSign  SampleTime=1/100
  VISUMatrixSignLights_HighwayOverhang_21 : Outport  Tag=outport/VisuMatrixSignLights  Port=2  SampleTime=1/100
  wires:
  VISUMatrixSign_Mux/1(MatrixSigns) -> VISUMatrixSign_HighwayOverhang_21/1
  VISUMatrixSignLights_Mux/1(VISUMatrixSignLights_HighwayOverhang_21) -> VISUMatrixSignLights_HighwayOverhang_21/1
  Ground_1/1 -> VISUMatrixSignLights_Mux/1(MatrixSign_11)
  Ground_2/1 -> VISUMatrixSignLights_Mux/2(MatrixSign_53)
  Ground_3/1 -> VISUMatrixSign_Mux/1(MatrixSign_11)
  Ground_4/1 -> VISUMatrixSign_Mux/2(MatrixSign_53)

== system TSR_Scenario_002_cs/HighwayOverhang_22 ==
  note: Resources
      |
      | 1: InformationSign\MatrixSign_GreenArrow.png: MatrixSign GreenArrow
      | 2: InformationSign\Empty.jpeg: Empty
      | 3: InformationSign\SEARCH_Logo.png: SEARCH Logo
      | 4: InformationSign\z274-50_black_full.png: z274-50 black full
      | 5: InformationSign\z274-51_black_full.png: z274-51 black full
      | 6: InformationSign\z274-52_black_full.png: z274-52 black full
      | 7: InformationSign\z274-53_black_full.png: z274-53 black full
      | 8: InformationSign\z274-54_black_full.png: z274-54 black full
      | 9: InformationSign\z274-55_black_full.png: z274-55 black full
      | 10: InformationSign\z274-56_black_full.png: z274-56 black full
      | 11: InformationSign\z274-57_black_full.png: z274-57 black full
      | 12: InformationSign\z274-58_black_full.png: z274-58 black full
      | 13: InformationSign\z274-59_black_full.png: z274-59 black full
      | 14: InformationSign\z274-60_black_full.png: z274-60 black full
      | 15: InformationSign\z274-61_black_full.png: z274-61 black full
      | 16: InformationSign\z274-62_black_full.png: z274-62 black full
      | 17: InformationSign\z274-63_black_full.png: z274-63 black full
  Ground_{1..4} (4 alike) : Ground
  VISUMatrixSignLights_Mux : Subsystem  Tag=mux/VisuMatrixSignLights  mask(PreScan User Interface: VisuMatrixSignLights){}
      mask help:
      | The VisuMatrixSignLights block provides a way to switch the lights on the matrix sign board on or off
      |
      | For more information, please click Help.
      mask Help: eval('openHelp(732)')
  VISUMatrixSign_Mux : Subsystem  Tag=mux/MatrixSign_v2  mask(PreScan User Interface: VisuMatrixSign){}
      mask help:
      | The VisuMatrixSign block provides a way to adapt the texture of the plates connected to an overhang, based on Resource IDs of the texture files.
      |
      | For more information, please click Help.
      settings: DeleteFcn=PreScanBlockDeleteFcn;
      mask Help: eval('openHelp(733)')
  VISUMatrixSign_HighwayOverhang_22 : Outport  Tag=outport/VisuMatrixSign  SampleTime=1/100
  VISUMatrixSignLights_HighwayOverhang_22 : Outport  Tag=outport/VisuMatrixSignLights  Port=2  SampleTime=1/100
  wires:
  VISUMatrixSign_Mux/1(MatrixSigns) -> VISUMatrixSign_HighwayOverhang_22/1
  VISUMatrixSignLights_Mux/1(VISUMatrixSignLights_HighwayOverhang_22) -> VISUMatrixSignLights_HighwayOverhang_22/1
  Ground_1/1 -> VISUMatrixSignLights_Mux/1(MatrixSign_35)
  Ground_2/1 -> VISUMatrixSignLights_Mux/2(MatrixSign_36)
  Ground_3/1 -> VISUMatrixSign_Mux/1(MatrixSign_35)
  Ground_4/1 -> VISUMatrixSign_Mux/2(MatrixSign_36)

== system TSR_Scenario_002_cs/HighwayOverhang_23 ==
  note: Resources
      |
      | 1: InformationSign\MatrixSign_GreenArrow.png: MatrixSign GreenArrow
      | 2: InformationSign\Empty.jpeg: Empty
      | 3: InformationSign\SEARCH_Logo.png: SEARCH Logo
      | 4: InformationSign\z274-50_black_full.png: z274-50 black full
      | 5: InformationSign\z274-51_black_full.png: z274-51 black full
      | 6: InformationSign\z274-52_black_full.png: z274-52 black full
      | 7: InformationSign\z274-53_black_full.png: z274-53 black full
      | 8: InformationSign\z274-54_black_full.png: z274-54 black full
      | 9: InformationSign\z274-55_black_full.png: z274-55 black full
      | 10: InformationSign\z274-56_black_full.png: z274-56 black full
      | 11: InformationSign\z274-57_black_full.png: z274-57 black full
      | 12: InformationSign\z274-58_black_full.png: z274-58 black full
      | 13: InformationSign\z274-59_black_full.png: z274-59 black full
      | 14: InformationSign\z274-60_black_full.png: z274-60 black full
      | 15: InformationSign\z274-61_black_full.png: z274-61 black full
      | 16: InformationSign\z274-62_black_full.png: z274-62 black full
      | 17: InformationSign\z274-63_black_full.png: z274-63 black full
  Ground_{1..4} (4 alike) : Ground
  VISUMatrixSignLights_Mux : Subsystem  Tag=mux/VisuMatrixSignLights  mask(PreScan User Interface: VisuMatrixSignLights){}
      mask help:
      | The VisuMatrixSignLights block provides a way to switch the lights on the matrix sign board on or off
      |
      | For more information, please click Help.
      mask Help: eval('openHelp(732)')
  VISUMatrixSign_Mux : Subsystem  Tag=mux/MatrixSign_v2  mask(PreScan User Interface: VisuMatrixSign){}
      mask help:
      | The VisuMatrixSign block provides a way to adapt the texture of the plates connected to an overhang, based on Resource IDs of the texture files.
      |
      | For more information, please click Help.
      settings: DeleteFcn=PreScanBlockDeleteFcn;
      mask Help: eval('openHelp(733)')
  VISUMatrixSign_HighwayOverhang_23 : Outport  Tag=outport/VisuMatrixSign  SampleTime=1/100
  VISUMatrixSignLights_HighwayOverhang_23 : Outport  Tag=outport/VisuMatrixSignLights  Port=2  SampleTime=1/100
  wires:
  VISUMatrixSign_Mux/1(MatrixSigns) -> VISUMatrixSign_HighwayOverhang_23/1
  VISUMatrixSignLights_Mux/1(VISUMatrixSignLights_HighwayOverhang_23) -> VISUMatrixSignLights_HighwayOverhang_23/1
  Ground_1/1 -> VISUMatrixSignLights_Mux/1(MatrixSign_13)
  Ground_2/1 -> VISUMatrixSignLights_Mux/2(MatrixSign_54)
  Ground_3/1 -> VISUMatrixSign_Mux/1(MatrixSign_13)
  Ground_4/1 -> VISUMatrixSign_Mux/2(MatrixSign_54)

== system TSR_Scenario_002_cs/HighwayOverhang_24 ==
  note: Resources
      |
      | 1: InformationSign\MatrixSign_GreenArrow.png: MatrixSign GreenArrow
      | 2: InformationSign\Empty.jpeg: Empty
      | 3: InformationSign\SEARCH_Logo.png: SEARCH Logo
      | 4: InformationSign\z274-50_black_full.png: z274-50 black full
      | 5: InformationSign\z274-51_black_full.png: z274-51 black full
      | 6: InformationSign\z274-52_black_full.png: z274-52 black full
      | 7: InformationSign\z274-53_black_full.png: z274-53 black full
      | 8: InformationSign\z274-54_black_full.png: z274-54 black full
      | 9: InformationSign\z274-55_black_full.png: z274-55 black full
      | 10: InformationSign\z274-56_black_full.png: z274-56 black full
      | 11: InformationSign\z274-57_black_full.png: z274-57 black full
      | 12: InformationSign\z274-58_black_full.png: z274-58 black full
      | 13: InformationSign\z274-59_black_full.png: z274-59 black full
      | 14: InformationSign\z274-60_black_full.png: z274-60 black full
      | 15: InformationSign\z274-61_black_full.png: z274-61 black full
      | 16: InformationSign\z274-62_black_full.png: z274-62 black full
      | 17: InformationSign\z274-63_black_full.png: z274-63 black full
  Ground_{1..4} (4 alike) : Ground
  VISUMatrixSignLights_Mux : Subsystem  Tag=mux/VisuMatrixSignLights  mask(PreScan User Interface: VisuMatrixSignLights){}
      mask help:
      | The VisuMatrixSignLights block provides a way to switch the lights on the matrix sign board on or off
      |
      | For more information, please click Help.
      mask Help: eval('openHelp(732)')
  VISUMatrixSign_Mux : Subsystem  Tag=mux/MatrixSign_v2  mask(PreScan User Interface: VisuMatrixSign){}
      mask help:
      | The VisuMatrixSign block provides a way to adapt the texture of the plates connected to an overhang, based on Resource IDs of the texture files.
      |
      | For more information, please click Help.
      settings: DeleteFcn=PreScanBlockDeleteFcn;
      mask Help: eval('openHelp(733)')
  VISUMatrixSign_HighwayOverhang_24 : Outport  Tag=outport/VisuMatrixSign  SampleTime=1/100
  VISUMatrixSignLights_HighwayOverhang_24 : Outport  Tag=outport/VisuMatrixSignLights  Port=2  SampleTime=1/100
  wires:
  VISUMatrixSign_Mux/1(MatrixSigns) -> VISUMatrixSign_HighwayOverhang_24/1
  VISUMatrixSignLights_Mux/1(VISUMatrixSignLights_HighwayOverhang_24) -> VISUMatrixSignLights_HighwayOverhang_24/1
  Ground_1/1 -> VISUMatrixSignLights_Mux/1(MatrixSign_25)
  Ground_2/1 -> VISUMatrixSignLights_Mux/2(MatrixSign_55)
  Ground_3/1 -> VISUMatrixSign_Mux/1(MatrixSign_25)
  Ground_4/1 -> VISUMatrixSign_Mux/2(MatrixSign_55)

== system TSR_Scenario_002_cs/HighwayOverhang_25 ==
  note: Resources
      |
      | 1: InformationSign\MatrixSign_GreenArrow.png: MatrixSign GreenArrow
      | 2: InformationSign\Empty.jpeg: Empty
      | 3: InformationSign\SEARCH_Logo.png: SEARCH Logo
      | 4: InformationSign\z274-50_black_full.png: z274-50 black full
      | 5: InformationSign\z274-51_black_full.png: z274-51 black full
      | 6: InformationSign\z274-52_black_full.png: z274-52 black full
      | 7: InformationSign\z274-53_black_full.png: z274-53 black full
      | 8: InformationSign\z274-54_black_full.png: z274-54 black full
      | 9: InformationSign\z274-55_black_full.png: z274-55 black full
      | 10: InformationSign\z274-56_black_full.png: z274-56 black full
      | 11: InformationSign\z274-57_black_full.png: z274-57 black full
      | 12: InformationSign\z274-58_black_full.png: z274-58 black full
      | 13: InformationSign\z274-59_black_full.png: z274-59 black full
      | 14: InformationSign\z274-60_black_full.png: z274-60 black full
      | 15: InformationSign\z274-61_black_full.png: z274-61 black full
      | 16: InformationSign\z274-62_black_full.png: z274-62 black full
      | 17: InformationSign\z274-63_black_full.png: z274-63 black full
  Ground_{1..4} (4 alike) : Ground
  VISUMatrixSignLights_Mux : Subsystem  Tag=mux/VisuMatrixSignLights  mask(PreScan User Interface: VisuMatrixSignLights){}
      mask help:
      | The VisuMatrixSignLights block provides a way to switch the lights on the matrix sign board on or off
      |
      | For more information, please click Help.
      mask Help: eval('openHelp(732)')
  VISUMatrixSign_Mux : Subsystem  Tag=mux/MatrixSign_v2  mask(PreScan User Interface: VisuMatrixSign){}
      mask help:
      | The VisuMatrixSign block provides a way to adapt the texture of the plates connected to an overhang, based on Resource IDs of the texture files.
      |
      | For more information, please click Help.
      settings: DeleteFcn=PreScanBlockDeleteFcn;
      mask Help: eval('openHelp(733)')
  VISUMatrixSign_HighwayOverhang_25 : Outport  Tag=outport/VisuMatrixSign  SampleTime=1/100
  VISUMatrixSignLights_HighwayOverhang_25 : Outport  Tag=outport/VisuMatrixSignLights  Port=2  SampleTime=1/100
  wires:
  VISUMatrixSign_Mux/1(MatrixSigns) -> VISUMatrixSign_HighwayOverhang_25/1
  VISUMatrixSignLights_Mux/1(VISUMatrixSignLights_HighwayOverhang_25) -> VISUMatrixSignLights_HighwayOverhang_25/1
  Ground_1/1 -> VISUMatrixSignLights_Mux/1(MatrixSign_26)
  Ground_2/1 -> VISUMatrixSignLights_Mux/2(MatrixSign_56)
  Ground_3/1 -> VISUMatrixSign_Mux/1(MatrixSign_26)
  Ground_4/1 -> VISUMatrixSign_Mux/2(MatrixSign_56)

== system TSR_Scenario_002_cs/HighwayOverhang_26 ==
  note: Resources
      |
      | 1: InformationSign\MatrixSign_GreenArrow.png: MatrixSign GreenArrow
      | 2: InformationSign\Empty.jpeg: Empty
      | 3: InformationSign\SEARCH_Logo.png: SEARCH Logo
      | 4: InformationSign\z274-50_black_full.png: z274-50 black full
      | 5: InformationSign\z274-51_black_full.png: z274-51 black full
      | 6: InformationSign\z274-52_black_full.png: z274-52 black full
      | 7: InformationSign\z274-53_black_full.png: z274-53 black full
      | 8: InformationSign\z274-54_black_full.png: z274-54 black full
      | 9: InformationSign\z274-55_black_full.png: z274-55 black full
      | 10: InformationSign\z274-56_black_full.png: z274-56 black full
      | 11: InformationSign\z274-57_black_full.png: z274-57 black full
      | 12: InformationSign\z274-58_black_full.png: z274-58 black full
      | 13: InformationSign\z274-59_black_full.png: z274-59 black full
      | 14: InformationSign\z274-60_black_full.png: z274-60 black full
      | 15: InformationSign\z274-61_black_full.png: z274-61 black full
      | 16: InformationSign\z274-62_black_full.png: z274-62 black full
      | 17: InformationSign\z274-63_black_full.png: z274-63 black full
  Ground_{1..4} (4 alike) : Ground
  VISUMatrixSignLights_Mux : Subsystem  Tag=mux/VisuMatrixSignLights  mask(PreScan User Interface: VisuMatrixSignLights){}
      mask help:
      | The VisuMatrixSignLights block provides a way to switch the lights on the matrix sign board on or off
      |
      | For more information, please click Help.
      mask Help: eval('openHelp(732)')
  VISUMatrixSign_Mux : Subsystem  Tag=mux/MatrixSign_v2  mask(PreScan User Interface: VisuMatrixSign){}
      mask help:
      | The VisuMatrixSign block provides a way to adapt the texture of the plates connected to an overhang, based on Resource IDs of the texture files.
      |
      | For more information, please click Help.
      settings: DeleteFcn=PreScanBlockDeleteFcn;
      mask Help: eval('openHelp(733)')
  VISUMatrixSign_HighwayOverhang_26 : Outport  Tag=outport/VisuMatrixSign  SampleTime=1/100
  VISUMatrixSignLights_HighwayOverhang_26 : Outport  Tag=outport/VisuMatrixSignLights  Port=2  SampleTime=1/100
  wires:
  VISUMatrixSign_Mux/1(MatrixSigns) -> VISUMatrixSign_HighwayOverhang_26/1
  VISUMatrixSignLights_Mux/1(VISUMatrixSignLights_HighwayOverhang_26) -> VISUMatrixSignLights_HighwayOverhang_26/1
  Ground_1/1 -> VISUMatrixSignLights_Mux/1(MatrixSign_37)
  Ground_2/1 -> VISUMatrixSignLights_Mux/2(MatrixSign_38)
  Ground_3/1 -> VISUMatrixSign_Mux/1(MatrixSign_37)
  Ground_4/1 -> VISUMatrixSign_Mux/2(MatrixSign_38)

== system TSR_Scenario_002_cs/HighwayOverhang_27 ==
  note: Resources
      |
      | 1: InformationSign\MatrixSign_GreenArrow.png: MatrixSign GreenArrow
      | 2: InformationSign\Empty.jpeg: Empty
      | 3: InformationSign\SEARCH_Logo.png: SEARCH Logo
      | 4: InformationSign\z274-50_black_full.png: z274-50 black full
      | 5: InformationSign\z274-51_black_full.png: z274-51 black full
      | 6: InformationSign\z274-52_black_full.png: z274-52 black full
      | 7: InformationSign\z274-53_black_full.png: z274-53 black full
      | 8: InformationSign\z274-54_black_full.png: z274-54 black full
      | 9: InformationSign\z274-55_black_full.png: z274-55 black full
      | 10: InformationSign\z274-56_black_full.png: z274-56 black full
      | 11: InformationSign\z274-57_black_full.png: z274-57 black full
      | 12: InformationSign\z274-58_black_full.png: z274-58 black full
      | 13: InformationSign\z274-59_black_full.png: z274-59 black full
      | 14: InformationSign\z274-60_black_full.png: z274-60 black full
      | 15: InformationSign\z274-61_black_full.png: z274-61 black full
      | 16: InformationSign\z274-62_black_full.png: z274-62 black full
      | 17: InformationSign\z274-63_black_full.png: z274-63 black full
  Ground_{1..4} (4 alike) : Ground
  VISUMatrixSignLights_Mux : Subsystem  Tag=mux/VisuMatrixSignLights  mask(PreScan User Interface: VisuMatrixSignLights){}
      mask help:
      | The VisuMatrixSignLights block provides a way to switch the lights on the matrix sign board on or off
      |
      | For more information, please click Help.
      mask Help: eval('openHelp(732)')
  VISUMatrixSign_Mux : Subsystem  Tag=mux/MatrixSign_v2  mask(PreScan User Interface: VisuMatrixSign){}
      mask help:
      | The VisuMatrixSign block provides a way to adapt the texture of the plates connected to an overhang, based on Resource IDs of the texture files.
      |
      | For more information, please click Help.
      settings: DeleteFcn=PreScanBlockDeleteFcn;
      mask Help: eval('openHelp(733)')
  VISUMatrixSign_HighwayOverhang_27 : Outport  Tag=outport/VisuMatrixSign  SampleTime=1/100
  VISUMatrixSignLights_HighwayOverhang_27 : Outport  Tag=outport/VisuMatrixSignLights  Port=2  SampleTime=1/100
  wires:
  VISUMatrixSign_Mux/1(MatrixSigns) -> VISUMatrixSign_HighwayOverhang_27/1
  VISUMatrixSignLights_Mux/1(VISUMatrixSignLights_HighwayOverhang_27) -> VISUMatrixSignLights_HighwayOverhang_27/1
  Ground_1/1 -> VISUMatrixSignLights_Mux/1(MatrixSign_39)
  Ground_2/1 -> VISUMatrixSignLights_Mux/2(MatrixSign_40)
  Ground_3/1 -> VISUMatrixSign_Mux/1(MatrixSign_39)
  Ground_4/1 -> VISUMatrixSign_Mux/2(MatrixSign_40)
